simulink model "LHC_18kW_v8"  (R2015a)
settings: Solver=ode15s  StartTime=0.0  StopTime=1e4  RelTol=1e-3
libraries: simCryogenics_lib x152, nesl_utility x108, fl_lib x15
(part 2 of 2)

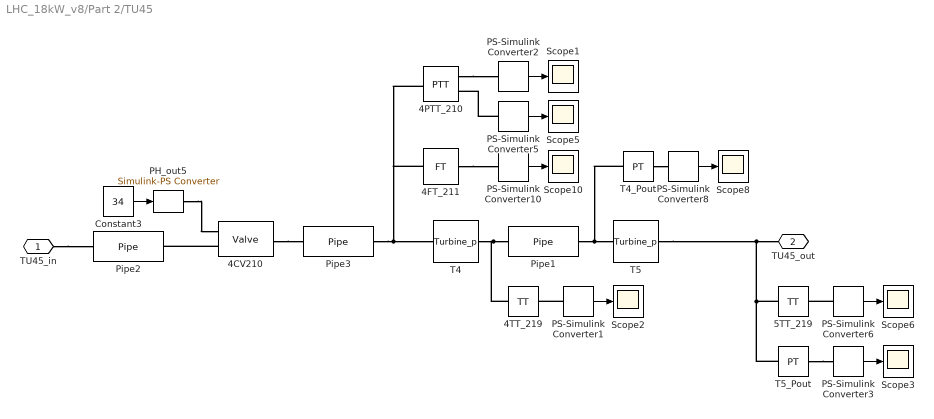
== system LHC_18kW_v8/Part 2/TU45 ==
  4CV210 : simCryogenics_lib/Elements/Valve  CVmax=75  ControlInputMin=0  ControlInputMax=100  Xt=0.65  Rv=50  lin_v=0  lim_v=0  K=2.4e-5 m^1.50000*kg^0.50000/s/bar^0.50000  Cmd_specify=off  Cmd_priority=High  Cmd=0  gamma_specify=off  gamma_priority=High  gamma=0  rho_specify=off  rho_priority=High  rho=0 kg/m^3  Xc_specify=off  Xc_priority=High  Xc=0  X_specify=off  X_priority=High  X=0  Y_specify=off  Y_priority=High  Y=0  CV_specify=off  CV_priority=High  CV=0
  4FT_211 : simCryogenics_lib/Sensors/FT
  4PTT_210 : simCryogenics_lib/Sensors/PTT
  4TT_219 : simCryogenics_lib/Sensors/TT
  5TT_219 : simCryogenics_lib/Sensors/TT
  Constant3 : Constant  Value=34
  PH_out5 : nesl_utility/Simulink-PS Converter  PhysicalDomain=network_engine_domain  SubClassName=ps_input  LeftPortType=input  RightPortType=output  PseudoPeriodic=off  Frequencies=[]  NoiseDistribution=none  NoiseParameters=[]  Unit=bar  AffineConversion=off  InputFiltering=off  SimscapeFilterOrder=1  InputFilterTimeConstant=0.001  UdotUserProvided=1
  PS-Simulink Converter{1..3,5..6,8,10} (7 alike) : nesl_utility/PS-Simulink Converter  PhysicalDomain=network_engine_domain  SubClassName=ps_output  LeftPortType=input  RightPortType=output  PseudoPeriodic=off  Frequencies=[]  Unit=1  AffineConversion=off
  Pipe1 : simCryogenics_lib/Elements/Pipe  Vol=0.01 m^3  Ideal=0  P0=7 bar  T0=64 K
  Pipe2 : simCryogenics_lib/Elements/Pipe  Vol=0.01 m^3  Ideal=0  P0=12 bar  T0=74 K
  Pipe3 : simCryogenics_lib/Elements/Pipe  Vol=0.01 m^3  Ideal=0  P0=11.5 bar  T0=74 K
  Scope{1..3,5..6,8,10} (7 alike) : Scope
      Scope1 settings: TimeRange=10000  SaveName=ScopeData7
      Scope10 settings: TimeRange=10000  SaveName=ScopeData9
      Scope2 settings: TimeRange=10000  SaveName=ScopeData58
      Scope3 settings: TimeRange=10000  SaveName=ScopeData60
      Scope5 settings: TimeRange=10000  SaveName=ScopeData16
      Scope6 settings: TimeRange=10000  SaveName=ScopeData35
      Scope8 settings: TimeRange=10000  SaveName=ScopeData59
  T4 : simCryogenics_lib/Elements/Turbine_p  A=1.2806e-04 m^2  D=0.0327 m  Mass=5.4 kg  cst_eff=0  eta0=0.79  Tin0=74 K  Pin0=11.2 bar  Pout0=7 bar  N0=1780 1/s  Q0=0 W  v0=0  I=0 kg*m^2  gamma_specify=off  gamma_priority=High  gamma=0  C_specify=off  C_priority=High  C=0  Z_specify=off  Z_priority=High  Z=0  Cp_specify=off  Cp_priority=High  Cp=0 kJ/kg/K  Sin_specify=off  Sin_priority=High  Sin=0 kJ/kg  T_specify=off  T_priority=High  T=0 K  HoutIs_specify=off  HoutIs_priority=High  HoutIs=0 kJ/kg  u1_specify=off  u1_priority=High  u1=0 m/s  c1_specify=off  c1_priority=High  c1=0 m/s  v_specify=off  v_priority=High  v=0  eta_specify=off  eta_priority=High  eta=0  eta_var_specify=off  eta_var_priority=High  eta_var=0  N_specify=off  N_priority=High  N=0 rad/s  Q_specify=off  Q_priority=High  Q=0 W
  T4_Pout : simCryogenics_lib/Sensors/PT
  T5 : simCryogenics_lib/Elements/Turbine_p  A=1.8991e-04 m^2  D=0.037 m  Mass=5.4 kg  cst_eff=0  eta0=0.79  Tin0=64 K  Pin0=7 bar  Pout0=2.92 bar  N0=1900 1/s  Q0=0 W  v0=0  I=0 kg*m^2  gamma_specify=off  gamma_priority=High  gamma=0  C_specify=off  C_priority=High  C=0  Z_specify=off  Z_priority=High  Z=0  Cp_specify=off  Cp_priority=High  Cp=0 kJ/kg/K  Sin_specify=off  Sin_priority=High  Sin=0 kJ/kg  T_specify=off  T_priority=High  T=0 K  HoutIs_specify=off  HoutIs_priority=High  HoutIs=0 kJ/kg  u1_specify=off  u1_priority=High  u1=0 m/s  c1_specify=off  c1_priority=High  c1=0 m/s  v_specify=off  v_priority=High  v=0  eta_specify=off  eta_priority=High  eta=0  eta_var_specify=off  eta_var_priority=High  eta_var=0  N_specify=off  N_priority=High  N=0 rad/s  Q_specify=off  Q_priority=High  Q=0 W
  T5_Pout : simCryogenics_lib/Sensors/PT
  TU45_in : PMIOPort  Port=1  Side=Left
  TU45_out : PMIOPort  Port=2  Side=Right
  wires:
  Constant3/1 -> PH_out5/1
  PS-Simulink Converter5/1 -> Scope5/1
  PS-Simulink Converter10/1 -> Scope10/1
  PS-Simulink Converter6/1 -> Scope6/1
  PS-Simulink Converter2/1 -> Scope1/1
  PS-Simulink Converter1/1 -> Scope2/1
  PS-Simulink Converter8/1 -> Scope8/1
  PS-Simulink Converter3/1 -> Scope3/1
  connections:
  4CV210/RConn1 -- Pipe3/LConn1
  PH_out5/RConn1 -- 4CV210/LConn1
  Pipe3/RConn1 -- 4FT_211/LConn1 -- 4PTT_210/LConn1 -- T4/LConn1
  T4/RConn1 -- 4TT_219/LConn1 -- Pipe1/LConn1
  TU45_in/RConn1 -- Pipe2/LConn1
  4CV210/LConn2 -- Pipe2/RConn1
  4FT_211/RConn1 -- PS-Simulink Converter10/LConn1
  PS-Simulink Converter5/LConn1 -- 4PTT_210/RConn2
  PS-Simulink Converter6/LConn1 -- 5TT_219/RConn1
  4PTT_210/RConn1 -- PS-Simulink Converter2/LConn1
  5TT_219/LConn1 -- T5/RConn1 -- TU45_out/RConn1 -- T5_Pout/LConn1
  Pipe1/RConn1 -- T4_Pout/LConn1 -- T5/LConn1
  PS-Simulink Converter1/LConn1 -- 4TT_219/RConn1
  T4_Pout/RConn1 -- PS-Simulink Converter8/LConn1
  T5_Pout/RConn1 -- PS-Simulink Converter3/LConn1

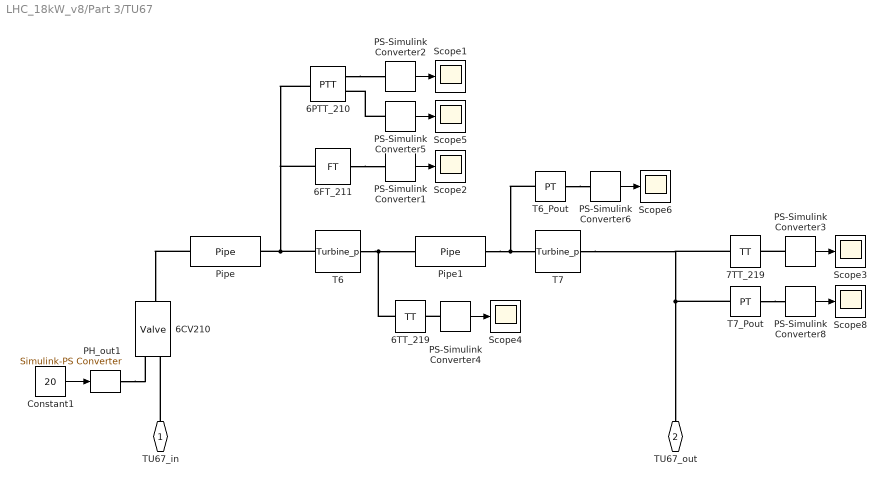
== system LHC_18kW_v8/Part 3/TU67 ==
  6CV210 : simCryogenics_lib/Elements/Valve  CVmax=58  ControlInputMin=0  ControlInputMax=100  Xt=0.65  Rv=50  lin_v=0  lim_v=0  K=2.4e-5 m^1.50000*kg^0.50000/s/bar^0.50000  Cmd_specify=off  Cmd_priority=High  Cmd=0  gamma_specify=off  gamma_priority=High  gamma=0  rho_specify=off  rho_priority=High  rho=0 kg/m^3  Xc_specify=off  Xc_priority=High  Xc=0  X_specify=off  X_priority=High  X=0  Y_specify=off  Y_priority=High  Y=0  CV_specify=off  CV_priority=High  CV=0
  6FT_211 : simCryogenics_lib/Sensors/FT
  6PTT_210 : simCryogenics_lib/Sensors/PTT
  6TT_219 : simCryogenics_lib/Sensors/TT
  7TT_219 : simCryogenics_lib/Sensors/TT
  Constant1 : Constant  Value=20
  PH_out1 : nesl_utility/Simulink-PS Converter  PhysicalDomain=network_engine_domain  SubClassName=ps_input  LeftPortType=input  RightPortType=output  PseudoPeriodic=off  Frequencies=[]  NoiseDistribution=none  NoiseParameters=[]  Unit=bar  AffineConversion=off  InputFiltering=off  SimscapeFilterOrder=1  InputFilterTimeConstant=0.001  UdotUserProvided=1
  PS-Simulink Converter{1..6,8} (7 alike) : nesl_utility/PS-Simulink Converter  PhysicalDomain=network_engine_domain  SubClassName=ps_output  LeftPortType=input  RightPortType=output  PseudoPeriodic=off  Frequencies=[]  Unit=1  AffineConversion=off
  Pipe : simCryogenics_lib/Elements/Pipe  Vol=0.01 m^3  Ideal=0  P0=13.5 bar  T0=37.3 K
  Pipe1 : simCryogenics_lib/Elements/Pipe  Vol=0.01 m^3  Ideal=0  P0=7.2 bar  T0=31.5 K
  Scope{1..6,8} (7 alike) : Scope
      Scope1 settings: TimeRange=10000  YMin=12.5  YMax=16.5  SaveName=ScopeData36
      Scope2 settings: TimeRange=10000  YMin=0.106  YMax=0.10925  SaveName=ScopeData37
      Scope3 settings: TimeRange=10000  YMin=100  YMax=180  SaveName=ScopeData26
      Scope4 settings: TimeRange=10000  YMin=100  YMax=180  SaveName=ScopeData61
      Scope5 settings: TimeRange=10000  YMin=34  YMax=40  SaveName=ScopeData43
      Scope6 settings: TimeRange=10000  SaveName=ScopeData62
      Scope8 settings: TimeRange=10000  SaveName=ScopeData27
  T6 : simCryogenics_lib/Elements/Turbine_p  A=3.5404e-05 m^2  D=0.0165 m  Mass=0.6 kg  cst_eff=0  eta0=0.74  Tin0=37.3 K  Pin0=12.9 bar  Pout0=7.17 bar  N0=2780 1/s  Q0=0 W  v0=0  I=0 kg*m^2  gamma_specify=off  gamma_priority=High  gamma=0  C_specify=off  C_priority=High  C=0  Z_specify=off  Z_priority=High  Z=0  Cp_specify=off  Cp_priority=High  Cp=0 kJ/kg/K  Sin_specify=off  Sin_priority=High  Sin=0 kJ/kg  T_specify=off  T_priority=High  T=0 K  HoutIs_specify=off  HoutIs_priority=High  HoutIs=0 kJ/kg  u1_specify=off  u1_priority=High  u1=0 m/s  c1_specify=off  c1_priority=High  c1=0 m/s  v_specify=off  v_priority=High  v=0  eta_specify=off  eta_priority=High  eta=0  eta_var_specify=off  eta_var_priority=High  eta_var=0  N_specify=off  N_priority=High  N=0 rad/s  Q_specify=off  Q_priority=High  Q=0 W
  T6_Pout : simCryogenics_lib/Sensors/PT
  T7 : simCryogenics_lib/Elements/Turbine_p  A=5.7857e-05 m^2  D=0.0209 m  Mass=1.8 kg  cst_eff=0  eta0=0.76  Tin0=31.5 K  Pin0=7.2 bar  Pout0=2.94 bar  N0=2400 1/s  Q0=0 W  v0=0  I=0 kg*m^2  gamma_specify=off  gamma_priority=High  gamma=0  C_specify=off  C_priority=High  C=0  Z_specify=off  Z_priority=High  Z=0  Cp_specify=off  Cp_priority=High  Cp=0 kJ/kg/K  Sin_specify=off  Sin_priority=High  Sin=0 kJ/kg  T_specify=off  T_priority=High  T=0 K  HoutIs_specify=off  HoutIs_priority=High  HoutIs=0 kJ/kg  u1_specify=off  u1_priority=High  u1=0 m/s  c1_specify=off  c1_priority=High  c1=0 m/s  v_specify=off  v_priority=High  v=0  eta_specify=off  eta_priority=High  eta=0  eta_var_specify=off  eta_var_priority=High  eta_var=0  N_specify=off  N_priority=High  N=0 rad/s  Q_specify=off  Q_priority=High  Q=0 W
  T7_Pout : simCryogenics_lib/Sensors/PT
  TU67_in : PMIOPort  Port=1  Side=Left
  TU67_out : PMIOPort  Port=2  Side=Right
  wires:
  Constant1/1 -> PH_out1/1
  PS-Simulink Converter5/1 -> Scope5/1
  PS-Simulink Converter1/1 -> Scope2/1
  PS-Simulink Converter3/1 -> Scope3/1
  PS-Simulink Converter8/1 -> Scope8/1
  PS-Simulink Converter2/1 -> Scope1/1
  PS-Simulink Converter4/1 -> Scope4/1
  PS-Simulink Converter6/1 -> Scope6/1
  connections:
  TU67_in/RConn1 -- 6CV210/LConn2
  PH_out1/RConn1 -- 6CV210/LConn1
  Pipe/LConn1 -- 6CV210/RConn1
  T6/LConn1 -- 6FT_211/LConn1 -- 6PTT_210/LConn1 -- Pipe/RConn1
  T7/RConn1 -- 7TT_219/LConn1 -- T7_Pout/LConn1 -- TU67_out/RConn1
  6FT_211/RConn1 -- PS-Simulink Converter1/LConn1
  PS-Simulink Converter5/LConn1 -- 6PTT_210/RConn2
  6PTT_210/RConn1 -- PS-Simulink Converter2/LConn1
  T7_Pout/RConn1 -- PS-Simulink Converter8/LConn1
  PS-Simulink Converter3/LConn1 -- 7TT_219/RConn1
  T6/RConn1 -- 6TT_219/LConn1 -- Pipe1/LConn1
  Pipe1/RConn1 -- T6_Pout/LConn1 -- T7/LConn1
  PS-Simulink Converter4/LConn1 -- 6TT_219/RConn1
  T6_Pout/RConn1 -- PS-Simulink Converter6/LConn1

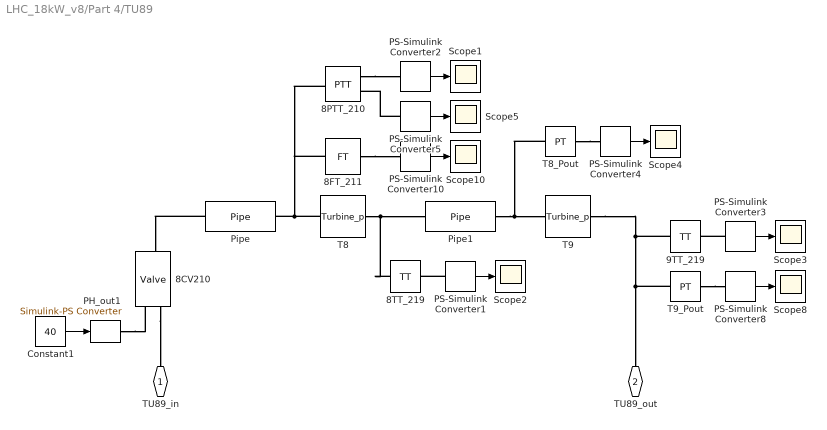
== system LHC_18kW_v8/Part 4/TU89 ==
  8CV210 : simCryogenics_lib/Elements/Valve  CVmax=37  ControlInputMin=0  ControlInputMax=100  Xt=0.65  Rv=50  lin_v=0  lim_v=0  K=2.4e-5 m^1.50000*kg^0.50000/s/bar^0.50000  Cmd_specify=off  Cmd_priority=High  Cmd=0  gamma_specify=off  gamma_priority=High  gamma=0  rho_specify=off  rho_priority=High  rho=0 kg/m^3  Xc_specify=off  Xc_priority=High  Xc=0  X_specify=off  X_priority=High  X=0  Y_specify=off  Y_priority=High  Y=0  CV_specify=off  CV_priority=High  CV=0
  8FT_211 : simCryogenics_lib/Sensors/FT
  8PTT_210 : simCryogenics_lib/Sensors/PTT
  8TT_219 : simCryogenics_lib/Sensors/TT
  9TT_219 : simCryogenics_lib/Sensors/TT
  Constant1 : Constant  Value=40
  PH_out1 : nesl_utility/Simulink-PS Converter  PhysicalDomain=network_engine_domain  SubClassName=ps_input  LeftPortType=input  RightPortType=output  PseudoPeriodic=off  Frequencies=[]  NoiseDistribution=none  NoiseParameters=[]  Unit=bar  AffineConversion=off  InputFiltering=off  SimscapeFilterOrder=1  InputFilterTimeConstant=0.001  UdotUserProvided=1
  PS-Simulink Converter{1..5,8,10} (7 alike) : nesl_utility/PS-Simulink Converter  PhysicalDomain=network_engine_domain  SubClassName=ps_output  LeftPortType=input  RightPortType=output  PseudoPeriodic=off  Frequencies=[]  Unit=1  AffineConversion=off
  Pipe : simCryogenics_lib/Elements/Pipe  Vol=0.01 m^3  Ideal=0  P0=13 bar  T0=19.6 K
  Pipe1 : simCryogenics_lib/Elements/Pipe  Vol=0.01 m^3  Ideal=0  P0=12.5 bar  T0=14.4 K
  Scope{1..5,8,10} (7 alike) : Scope
      Scope1 settings: TimeRange=10000  YMin=12.7  YMax=12.975  SaveName=ScopeData32
      Scope10 settings: TimeRange=10000  SaveName=ScopeData34
      Scope2 settings: TimeRange=10000  YMin=100  YMax=180  SaveName=ScopeData63
      Scope3 settings: TimeRange=10000  YMin=100  YMax=180  SaveName=ScopeData45
      Scope4 settings: TimeRange=10000  SaveName=ScopeData64
      Scope5 settings: TimeRange=10000  YMin=20.2  YMax=21.4  SaveName=ScopeData33
      Scope8 settings: TimeRange=10000  SaveName=ScopeData46
  T8 : simCryogenics_lib/Elements/Turbine_p  A=5.8341e-05 m^2  D=0.020 m  Mass=10 kg  cst_eff=0  eta0=0.76  Tin0=19.6 K  Pin0=12.8 bar  Pout0=3.76 bar  N0=2200 1/s  Q0=0 W  v0=0  I=0 kg*m^2  gamma_specify=off  gamma_priority=High  gamma=0  C_specify=off  C_priority=High  C=0  Z_specify=off  Z_priority=High  Z=0  Cp_specify=off  Cp_priority=High  Cp=0 kJ/kg/K  Sin_specify=off  Sin_priority=High  Sin=0 kJ/kg  T_specify=off  T_priority=High  T=0 K  HoutIs_specify=off  HoutIs_priority=High  HoutIs=0 kJ/kg  u1_specify=off  u1_priority=High  u1=0 m/s  c1_specify=off  c1_priority=High  c1=0 m/s  v_specify=off  v_priority=High  v=0  eta_specify=off  eta_priority=High  eta=0  eta_var_specify=off  eta_var_priority=High  eta_var=0  N_specify=off  N_priority=High  N=0 rad/s  Q_specify=off  Q_priority=High  Q=0 W
  T8_Pout : simCryogenics_lib/Sensors/PT
  T9 : simCryogenics_lib/Elements/Turbine_p  A=1.3750e-04 m^2  D=0.0283 m  Mass=10 kg  cst_eff=0  eta0=0.79  Tin0=14.4 K  Pin0=4.6 bar  Pout0=1.21 bar  N0=1367 1/s  Q0=0 W  v0=0  I=0 kg*m^2  gamma_specify=off  gamma_priority=High  gamma=0  C_specify=off  C_priority=High  C=0  Z_specify=off  Z_priority=High  Z=0  Cp_specify=off  Cp_priority=High  Cp=0 kJ/kg/K  Sin_specify=off  Sin_priority=High  Sin=0 kJ/kg  T_specify=off  T_priority=High  T=0 K  HoutIs_specify=off  HoutIs_priority=High  HoutIs=0 kJ/kg  u1_specify=off  u1_priority=High  u1=0 m/s  c1_specify=off  c1_priority=High  c1=0 m/s  v_specify=off  v_priority=High  v=0  eta_specify=off  eta_priority=High  eta=0  eta_var_specify=off  eta_var_priority=High  eta_var=0  N_specify=off  N_priority=High  N=0 rad/s  Q_specify=off  Q_priority=High  Q=0 W
  T9_Pout : simCryogenics_lib/Sensors/PT
  TU89_in : PMIOPort  Port=1  Side=Left
  TU89_out : PMIOPort  Port=2  Side=Right
  wires:
  Constant1/1 -> PH_out1/1
  PS-Simulink Converter5/1 -> Scope5/1
  PS-Simulink Converter10/1 -> Scope10/1
  PS-Simulink Converter2/1 -> Scope1/1
  PS-Simulink Converter3/1 -> Scope3/1
  PS-Simulink Converter8/1 -> Scope8/1
  PS-Simulink Converter1/1 -> Scope2/1
  PS-Simulink Converter4/1 -> Scope4/1
  connections:
  PH_out1/RConn1 -- 8CV210/LConn1
  8CV210/LConn2 -- TU89_in/RConn1
  T8/LConn1 -- 8FT_211/LConn1 -- 8PTT_210/LConn1 -- Pipe/RConn1
  Pipe/LConn1 -- 8CV210/RConn1
  9TT_219/LConn1 -- T9/RConn1 -- T9_Pout/LConn1 -- TU89_out/RConn1
  8PTT_210/RConn1 -- PS-Simulink Converter2/LConn1
  PS-Simulink Converter5/LConn1 -- 8PTT_210/RConn2
  8FT_211/RConn1 -- PS-Simulink Converter10/LConn1
  T9_Pout/RConn1 -- PS-Simulink Converter8/LConn1
  PS-Simulink Converter3/LConn1 -- 9TT_219/RConn1
  T8/RConn1 -- 8TT_219/LConn1 -- Pipe1/LConn1
  Pipe1/RConn1 -- T8_Pout/LConn1 -- T9/LConn1
  PS-Simulink Converter1/LConn1 -- 8TT_219/RConn1
  T8_Pout/RConn1 -- PS-Simulink Converter4/LConn1

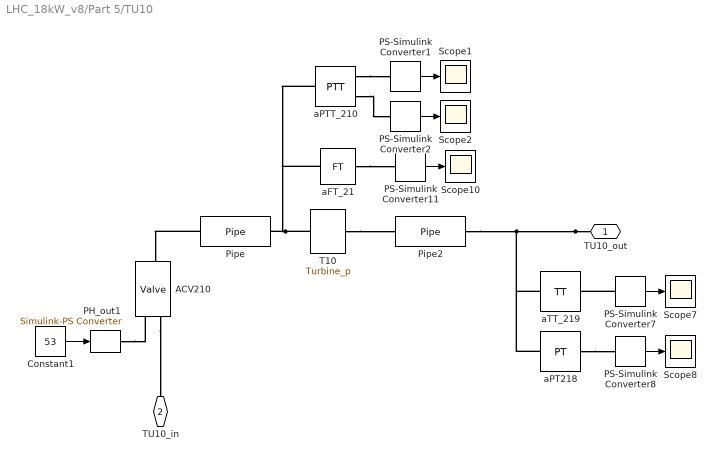
== system LHC_18kW_v8/Part 5/TU10 ==
  ACV210 : simCryogenics_lib/Elements/Valve  CVmax=11  ControlInputMin=0  ControlInputMax=100  Xt=0.65  Rv=50  lin_v=0  lim_v=0  K=2.4e-5 m^1.50000*kg^0.50000/s/bar^0.50000  Cmd_specify=off  Cmd_priority=High  Cmd=0  gamma_specify=off  gamma_priority=High  gamma=0  rho_specify=off  rho_priority=High  rho=0 kg/m^3  Xc_specify=off  Xc_priority=High  Xc=0  X_specify=off  X_priority=High  X=0  Y_specify=off  Y_priority=High  Y=0  CV_specify=off  CV_priority=High  CV=0
  Constant1 : Constant  Value=53
  PH_out1 : nesl_utility/Simulink-PS Converter  PhysicalDomain=network_engine_domain  SubClassName=ps_input  LeftPortType=input  RightPortType=output  PseudoPeriodic=off  Frequencies=[]  NoiseDistribution=none  NoiseParameters=[]  Unit=bar  AffineConversion=off  InputFiltering=off  SimscapeFilterOrder=1  InputFilterTimeConstant=0.001  UdotUserProvided=1
  PS-Simulink Converter{1..2,7..8,11} (5 alike) : nesl_utility/PS-Simulink Converter  PhysicalDomain=network_engine_domain  SubClassName=ps_output  LeftPortType=input  RightPortType=output  PseudoPeriodic=off  Frequencies=[]  Unit=1  AffineConversion=off
  Pipe : simCryogenics_lib/Elements/Pipe  Vol=0.01 m^3  Ideal=0  P0=13 bar  T0=8.1 K
  Pipe2 : simCryogenics_lib/Elements/Pipe  Vol=0.01 m^3  Ideal=0  P0=2.5 bar  T0=8.1 K
  Scope{1..2,7..8,10} (5 alike) : Scope
      Scope1 settings: TimeRange=233  YMin=3.0525  YMax=3.1075  SaveName=ScopeData5
      Scope10 settings: TimeRange=10000  SaveName=ScopeData52
      Scope2 settings: TimeRange=233  YMin=4.5004  YMax=4.501  SaveName=ScopeData13
      Scope7 settings: TimeRange=10000  SaveName=ScopeData53
      Scope8 settings: TimeRange=10000  SaveName=ScopeData54
  T10 : simCryogenics_lib/Elements/Turbine_p  A=3.1203e-05 m^2  D=0.0137 m  Mass=1.8 kg  cst_eff=0  eta0=0.72  Tin0=8.1 K  Pin0=12.8 bar  Pout0=2.98 bar  N0=1690 1/s  Q0=0 W  v0=0  I=0 kg*m^2  gamma_specify=off  gamma_priority=High  gamma=0  C_specify=off  C_priority=High  C=0  Z_specify=off  Z_priority=High  Z=0  Cp_specify=off  Cp_priority=High  Cp=0 kJ/kg/K  Sin_specify=off  Sin_priority=High  Sin=0 kJ/kg  T_specify=off  T_priority=High  T=0 K  HoutIs_specify=off  HoutIs_priority=High  HoutIs=0 kJ/kg  u1_specify=off  u1_priority=High  u1=0 m/s  c1_specify=off  c1_priority=High  c1=0 m/s  v_specify=off  v_priority=High  v=0  eta_specify=off  eta_priority=High  eta=0  eta_var_specify=off  eta_var_priority=High  eta_var=0  N_specify=off  N_priority=High  N=0 rad/s  Q_specify=off  Q_priority=High  Q=0 W
  aFT_21 : simCryogenics_lib/Sensors/FT
  aPT218 : simCryogenics_lib/Sensors/PT
  aPTT_210 : simCryogenics_lib/Sensors/PTT
  aTT_219 : simCryogenics_lib/Sensors/TT
  TU10_out : PMIOPort  Port=1  Side=Right
  TU10_in : PMIOPort  Port=2  Side=Left
  wires:
  PS-Simulink Converter8/1 -> Scope8/1
  PS-Simulink Converter7/1 -> Scope7/1
  PS-Simulink Converter11/1 -> Scope10/1
  PS-Simulink Converter1/1 -> Scope1/1
  PS-Simulink Converter2/1 -> Scope2/1
  Constant1/1 -> PH_out1/1
  connections:
  PS-Simulink Converter7/LConn1 -- aTT_219/RConn1
  aPT218/RConn1 -- PS-Simulink Converter8/LConn1
  aFT_21/RConn1 -- PS-Simulink Converter11/LConn1
  aPTT_210/RConn1 -- PS-Simulink Converter1/LConn1
  aPTT_210/RConn2 -- PS-Simulink Converter2/LConn1
  PH_out1/RConn1 -- ACV210/LConn1
  Pipe/LConn1 -- ACV210/RConn1
  T10/RConn1 -- Pipe2/LConn1
  TU10_out/RConn1 -- aTT_219/LConn1 -- aPT218/LConn1 -- Pipe2/RConn1
  ACV210/LConn2 -- TU10_in/RConn1
  Pipe/RConn1 -- aPTT_210/LConn1 -- aFT_21/LConn1 -- T10/LConn1

== system LHC_18kW_v8/Part 5/ctrl_TU10 ==
  Constant1 : Constant  Value=2.7
  Constant3 : Constant  Value=55
  PH_out1 : nesl_utility/Simulink-PS Converter  PhysicalDomain=network_engine_domain  SubClassName=ps_input  LeftPortType=input  RightPortType=output  PseudoPeriodic=off  Frequencies=[]  NoiseDistribution=none  NoiseParameters=[]  Unit=bar  AffineConversion=off  InputFiltering=on  SimscapeFilterOrder=1  InputFilterTimeConstant=0.001  UdotUserProvided=1
  PH_out3 : nesl_utility/Simulink-PS Converter  PhysicalDomain=network_engine_domain  SubClassName=ps_input  LeftPortType=input  RightPortType=output  PseudoPeriodic=off  Frequencies=[]  NoiseDistribution=none  NoiseParameters=[]  Unit=bar  AffineConversion=off  InputFiltering=on  SimscapeFilterOrder=1  InputFilterTimeConstant=0.001  UdotUserProvided=1
  PS Add : fl_lib/Physical Signals/Functions/PS Add
  PS Gain : fl_lib/Physical Signals/Functions/PS Gain  gain=100
  PS Subtract : fl_lib/Physical Signals/Functions/PS Subtract
  T6_Pout : simCryogenics_lib/Sensors/PT
  ctrl_TU10_out : PMIOPort  Port=1  Side=Right
  ctrl_TU10_in : PMIOPort  Port=2  Side=Left
  wires:
  Constant3/1 -> PH_out3/1
  Constant1/1 -> PH_out1/1
  connections:
  T6_Pout/LConn1 -- ctrl_TU10_in/RConn1
  T6_Pout/RConn1 -- PS Subtract/LConn1
  PS Add/LConn1 -- PS Gain/RConn1
  PS Add/LConn2 -- PH_out3/RConn1
  PH_out1/RConn1 -- PS Subtract/LConn2
  ctrl_TU10_out/RConn1 -- PS Add/RConn1
  PS Gain/LConn1 -- PS Subtract/RConn1
